simulink model "FAT_low_highF"  (R2021b)
settings: Solver=ode5  StartTime=0.0  StopTime=5  FixedStep=0.001  RelTol=1e-3
settings Model: Creator=admin  LastModifiedBy=ASUS
settings SolverCC: AlgebraicLoopSolver=TrustRegion
settings DataIOCC: SaveFormat=StructureWithTime
settings OptimizationCC: LifeSpan=inf
settings DebuggingCC: SFExecutionAtInitializationDiag=none  SFMachineParentedDataDiag=warning  ArithmeticOperatorsInVariantConditions=warning
settings HardwareCC: ProdBitPerSizeT=32  ProdBitPerPtrDiffT=32  ProdWordSize=32  ProdHWDeviceType=Specified
settings SFSimCC: CustomCodeUndefinedFunction=UseInterfaceOnly
settings CodeAppCC: StateflowObjectComments=on

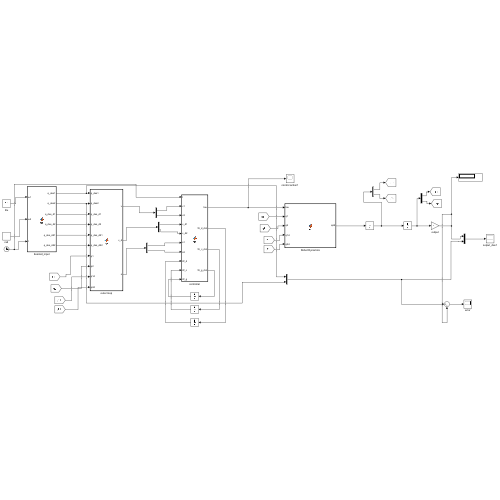
[thumbnail: Simulink's stored preview of the top-level diagram]
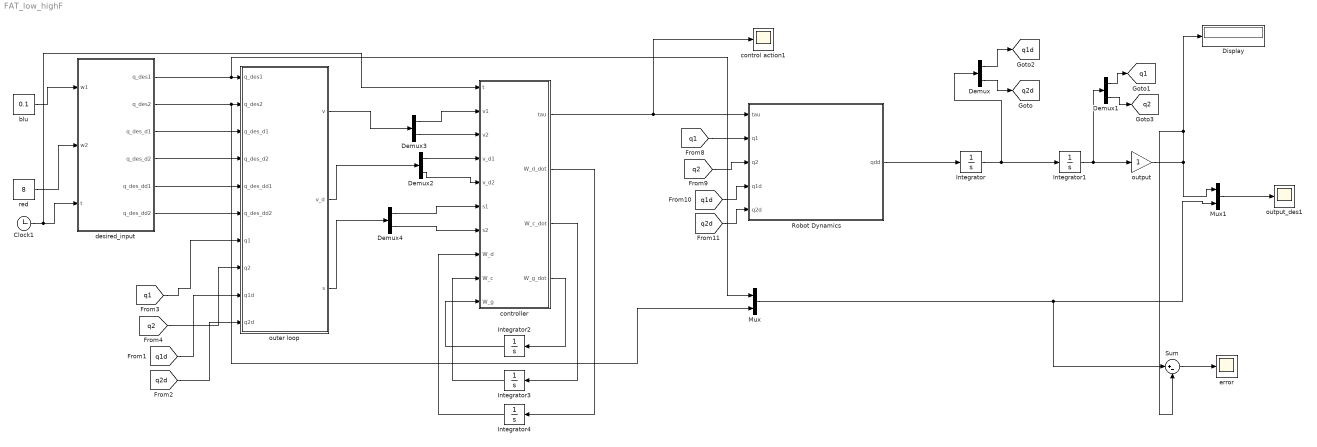
== system FAT_low_highF ==
  Clock1 : Clock
  Demux{,1..4} (5 alike) : Demux  Outputs=2
  Display : Display
  Integrator : Integrator  InitialCondition=[0;0]
  Integrator1 : Integrator  InitialCondition=[0;0]
  Integrator2 : Integrator  InitialCondition=rand(3,2)
  Integrator3 : Integrator  InitialCondition=rand(6,2)
  Integrator4 : Integrator  InitialCondition=rand(6,2)
  Mux : Mux  Inputs=2
  Mux1 : Mux  Inputs=2
  Robot Dynamics : MATLAB Function  TreatAsAtomicUnit=on
  Sum : Sum  Inputs=|+-
  blu : Constant  Value=0.1
  control action1 : Scope
  controller : MATLAB Function  TreatAsAtomicUnit=on
  desired_input : MATLAB Function  TreatAsAtomicUnit=on
  error : Scope
  outer loop : MATLAB Function  TreatAsAtomicUnit=on
  output : Gain
  output_des1 : Scope
  red : Constant  Value=8
  tag scope: q1=global, q1d=global, q2=global, q2d=global
  wires:
  [q2] -> Robot Dynamics/3(q2)
  [q1d] -> Robot Dynamics/4(q1d)
  [q1] -> Robot Dynamics/2(q1)
  [q2d] -> Robot Dynamics/5(q2d)
  Integrator/1 -> Demux/1, Integrator1/1
  output/1 -> Sum/2, Display/1, Mux1/1
  Demux1/1 -> [q1]
  Integrator1/1 -> Demux1/1, output/1
  Robot Dynamics/1(qdd) -> Integrator/1
  Demux/2 -> [q2d]
  Demux1/2 -> [q2]
  Demux/1 -> [q1d]
  controller/1(tau) -> control action1/1, Robot Dynamics/1(tau)
  controller/4(W_g_dot) -> Integrator2/1
  controller/3(W_c_dot) -> Integrator3/1
  controller/2(W_d_dot) -> Integrator4/1
  Integrator4/1 -> controller/8(W_d)
  Integrator3/1 -> controller/9(W_c)
  Integrator2/1 -> controller/10(W_g)
  [q1] -> outer loop/7(q1)
  [q2] -> outer loop/8(q2)
  [q1d] -> outer loop/9(q1d)
  [q2d] -> outer loop/10(q2d)
  outer loop/2(v_d) -> Demux2/1
  Demux2/1 -> controller/4(v_d1)
  Demux2/2 -> controller/5(v_d2)
  outer loop/1(v) -> Demux3/1
  Demux3/1 -> controller/2(v1)
  Demux3/2 -> controller/3(v2)
  outer loop/3(s) -> Demux4/1
  Demux4/1 -> controller/6(s1)
  Demux4/2 -> controller/7(s2)
  Mux/1 -> Sum/1, Mux1/2
  desired_input/1(q_des1) -> Mux/1, outer loop/1(q_des1)
  desired_input/2(q_des2) -> Mux/2, outer loop/2(q_des2)
  desired_input/3(q_des_d1) -> outer loop/3(q_des_d1)
  desired_input/4(q_des_d2) -> outer loop/4(q_des_d2)
  desired_input/5(q_des_dd1) -> outer loop/5(q_des_dd1)
  desired_input/6(q_des_dd2) -> outer loop/6(q_des_dd2)
  blu/1 -> desired_input/1(w1)
  red/1 -> desired_input/2(w2)
  Clock1/1 -> controller/1(t), desired_input/3(t)
  Sum/1 -> error/1
  Mux1/1 -> output_des1/1

== matlab function FAT_low_highF/Robot Dynamics ==
  data: tau input; q1 input; qdd output; q2 input; q1d input; q2d input
function qdd = fcn(tau,q1,q2,q1d,q2d)

% q1=q(1);
% q2=q(2);
% 
% q1d=qd(1);
% q2d=qd(2);

qd = [q1d;q2d];

m1=.1;
m2=.1;

I1=.01;
I2=.01;

l1=.12;
l2=.1;

lc1=l1/2;
lc2=l2/2;


g=9.8;



d11=m1*lc1^2+m2*(l1^2+lc2^2+2*l1*lc2^2+2*l1*l2*cos(q2))+I1+I2;
d12=m2*(lc2^2+l1*l2*cos(q2))+I2;
d22=m2*lc2^2+I2;

h=-m2*l1*lc2*sin(q2);

c121=h;
c211=h;
c112=-h;
c221=h;



M=[d11,d12;d12,d22];
C=[c121*q2d,c211*q1d+c221*q2d;c112*q1d,0];
G=[(m1*lc1+m2*l1)*g*cos(q1)+m2*lc2*g*cos(q1+q2);m2*lc2*cos(q1+q2)];


qdd=pinv(M)*((tau)-C*qd-G);

== matlab function FAT_low_highF/controller ==
  data: t input; tau output; v1 input; v2 input; v_d1 input; v_d2 input; s1 input; s2 input; W_d input; W_c input; W_g input; W_d_dot output; W_c_dot output; W_g_dot output
function [tau,W_d_dot,W_c_dot,W_g_dot] = fcn(t,v1,v2,v_d1,v_d2,s1,s2,W_d,W_c,W_g)
s = [s1;s2];
v = [v1;v2];
v_d = [v_d1;v_d2];
fn = 5;
%sinwt w =50
zz = [1;sin(fn*t);sin(2*fn*t)];

Zd = [zz,zeros(3,1);zeros(3,1),zz];

Zc = Zd;
Zg = zz;

D_hat = W_d'*Zd;
C_hat = W_c'*Zc;
g_hat = W_g'*Zg;

Qd = 1000*eye(6);
Qc = 1000*eye(6);
Qg = 1000*eye(3);

Kd = [8 0;0 8];
robust = [sign(s(1,1));sign(s(2,1))];
tau = g_hat+D_hat*v_d+C_hat*v-Kd*s-0.001*robust;
W_d_dot= -pinv(Qd)*Zd*s*v_d';
W_c_dot= -pinv(Qc)*Zc*s*v';
W_g_dot= -pinv(Qg)*Zg*s';

== matlab function FAT_low_highF/outer loop ==
  data: q_des1 input; v output; q_des2 input; q_des_d1 input; q_des_d2 input; q_des_dd1 input; q_des_dd2 input; q1 input; q2 input; q1d input; q2d input; v_d output; s output
function [v,v_d,s] = fcn(q_des1,q_des2,q_des_d1,q_des_d2,q_des_dd1,q_des_dd2,q1,q2,q1d,q2d)
gamma = 20;
q_des = [q_des1;q_des2];
q_des_d = [q_des_d1;q_des_d2];
q_des_dd = [q_des_dd1;q_des_dd2];
q = [q1;q2];
qd = [q1d;q2d];

e = q-q_des;
e_d = qd-q_des_d;

s = e_d+gamma*e;
v = q_des_d-gamma*e;
v_d = q_des_dd-gamma*e_d;

== matlab function FAT_low_highF/desired_input ==
  data: w1 input; q_des1 output; w2 input; q_des2 output; q_des_d1 output; q_des_d2 output; q_des_dd1 output; q_des_dd2 output; t input
function [q_des1,q_des2,q_des_d1,q_des_d2,q_des_dd1,q_des_dd2] = fcn(w1,w2,t)
q_des1 = sin(w1*t);
q_des2 = sin(w2*t);

q_des_d1 = w1*(cos(w1*t));
q_des_d2 = w2*(cos(w2*t));

q_des_dd1 = -w1^2*(sin(w1*t));
q_des_dd2 = -w2^2*(sin(w2*t));
